simulink model "gimbal_dynamic_identification_301019"  (R2018b)
settings: Solver=FixedStepAuto  StartTime=0.0  StopTime=100  FixedStep=0.01  RelTol=1e-3
values from neighbouring files (symbols this model uses):
  DIM = data{4}    [gimbal_dynamics.m]
  DIS = data{5}    [gimbal_dynamics.m]
  I1 = data{1}    [gimbal_dynamics.m]    (also in macierze_inercji.m = sym('I1', [4 4]))
  I2 = data{2}    [gimbal_dynamics.m]    (also in macierze_inercji.m = sym('I2', [4 4]))
  I3 = data{3}    [gimbal_dynamics.m]    (also in macierze_inercji.m = sym('I3', [4 4]))
  M = [ud_ucz(3:p-1) ud_ucz(3:p-1).^2 ud_ucz(3:p-1).^3 ud_ucz(2:p-2) ud_ucz(2:p-2).^2 ud_ucz(2:p-2).^3 ud_ucz(1:p-3) ud_ucz(1:p-3).^2 ud_ucz(1:p-3).^3 yd_ucz(3:p-1) yd_ucz(3:p-1).^2 yd_ucz(3:p-1).^3 yd_ucz(2:p-2) yd_ucz(2:p-2).^2 yd_ucz(2:p-2).^3 yd_ucz(1:p-3) yd_ucz(1:p-3).^2 yd_ucz(1:p-3).^3]    [Identification_20191023.m]    (also in MI_beta.m = fillmissing(M,'spline'); gimbal_dynamics.m = data{6}; macierze_inercji.m = sym('M', [1 3]))
libraries: simulink x4, simulink_extras x3
settings Model: Creator=Paweł Tymiński  LastModifiedBy=Paweł Tymiński
settings SolverCC: ZeroCrossAlgorithm=Adaptive
settings DebuggingCC: IgnoredZcDiagnostic=none
settings SFSimCC: SimUseLocalCustomCode=off
settings RTWCC: RTWUseLocalCustomCode=off
settings CodeAppCC: StateflowObjectComments=on
settings SimscapeCC: SimscapeNormalizeSystem=off

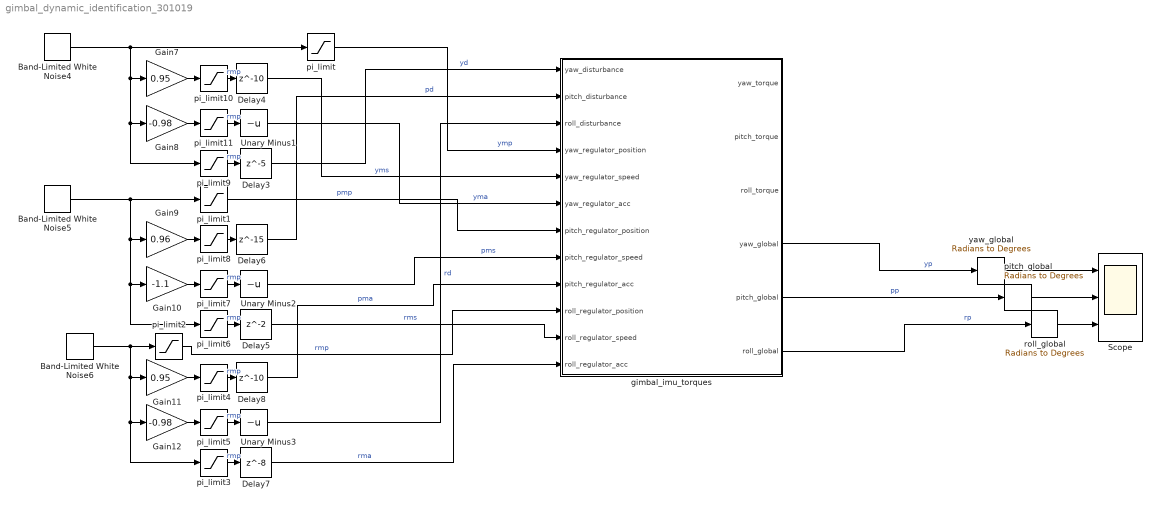
== system gimbal_dynamic_identification_301019 ==
  Band-Limited White Noise4 : simulink/Sources/Band-Limited White Noise  Cov=[0.02]  Ts=0.01  seed=[911]
  Band-Limited White Noise5 : simulink/Sources/Band-Limited White Noise  Cov=[0.015]  Ts=0.01  seed=[2137]
  Band-Limited White Noise6 : simulink/Sources/Band-Limited White Noise  Cov=[0.025]  Ts=0.01  seed=[1488]
  Delay3 : Delay  DelayLength=5  InitialCondition=0
  Delay4 : Delay  DelayLength=10  InitialCondition=0
  Delay5 : Delay  InitialCondition=0
  Delay6 : Delay  DelayLength=15  InitialCondition=0
  Delay7 : Delay  DelayLength=8  InitialCondition=0
  Delay8 : Delay  DelayLength=10  InitialCondition=0
  Gain10 : Gain  Gain=-1.1
  Gain11 : Gain  Gain=0.95
  Gain12 : Gain  Gain=-0.98
  Gain7 : Gain  Gain=0.95
  Gain8 : Gain  Gain=-0.98
  Gain9 : Gain  Gain=0.96
  Scope : Scope  NumInputPorts=3
  Unary Minus1 : UnaryMinus
  Unary Minus2 : UnaryMinus
  Unary Minus3 : UnaryMinus
  gimbal_imu_torques : Subsystem
  pi_limit{,1..11} (12 alike) : Saturate  UpperLimit=pi()  LowerLimit=-pi()
  pitch_global : simulink_extras/Transformations/Radians to Degrees
  roll_global : simulink_extras/Transformations/Radians to Degrees
  yaw_global : simulink_extras/Transformations/Radians to Degrees
  wires:
  gimbal_imu_torques/5(pitch_global) -> pitch_global/1  "pp"
  gimbal_imu_torques/4(yaw_global) -> yaw_global/1  "yp"
  gimbal_imu_torques/6(roll_global) -> roll_global/1  "rp"
  roll_global/1 -> Scope/3
  pitch_global/1 -> Scope/2
  yaw_global/1 -> Scope/1
  pi_limit/1 -> gimbal_imu_torques/4(yaw_regulator_position)  "ymp"
  Delay4/1 -> gimbal_imu_torques/5(yaw_regulator_speed)  "yms"
  pi_limit2/1 -> gimbal_imu_torques/10(roll_regulator_position)  "rmp"
  Unary Minus1/1 -> gimbal_imu_torques/6(yaw_regulator_acc)  "yma"
  Delay8/1 -> gimbal_imu_torques/9(pitch_regulator_acc)  "pma"
  pi_limit1/1 -> gimbal_imu_torques/7(pitch_regulator_position)  "pmp"
  Delay5/1 -> gimbal_imu_torques/11(roll_regulator_speed)  "rms"
  Unary Minus2/1 -> gimbal_imu_torques/8(pitch_regulator_speed)  "pms"
  Delay7/1 -> gimbal_imu_torques/12(roll_regulator_acc)  "rma"
  Band-Limited White Noise4/1 -> pi_limit9/1, Gain8/1, Gain7/1, pi_limit/1
  Band-Limited White Noise5/1 -> pi_limit6/1, Gain10/1, Gain9/1, pi_limit1/1
  Gain11/1 -> pi_limit4/1
  Gain8/1 -> pi_limit11/1
  Gain7/1 -> pi_limit10/1
  Band-Limited White Noise6/1 -> pi_limit3/1, Gain12/1, Gain11/1, pi_limit2/1
  Gain10/1 -> pi_limit7/1
  pi_limit8/1 -> Delay6/1
  Delay3/1 -> gimbal_imu_torques/1(yaw_disturbance)  "yd"
  Delay6/1 -> gimbal_imu_torques/2(pitch_disturbance)  "pd"
  Unary Minus3/1 -> gimbal_imu_torques/3(roll_disturbance)  "rd"
  pi_limit3/1 -> Delay7/1  "rmp"
  pi_limit4/1 -> Delay8/1  "rmp"
  Gain12/1 -> pi_limit5/1
  pi_limit5/1 -> Unary Minus3/1  "rmp"
  pi_limit6/1 -> Delay5/1  "rmp"
  pi_limit7/1 -> Unary Minus2/1  "rmp"
  Gain9/1 -> pi_limit8/1
  pi_limit9/1 -> Delay3/1  "rmp"
  pi_limit10/1 -> Delay4/1  "rmp"
  pi_limit11/1 -> Unary Minus1/1  "rmp"

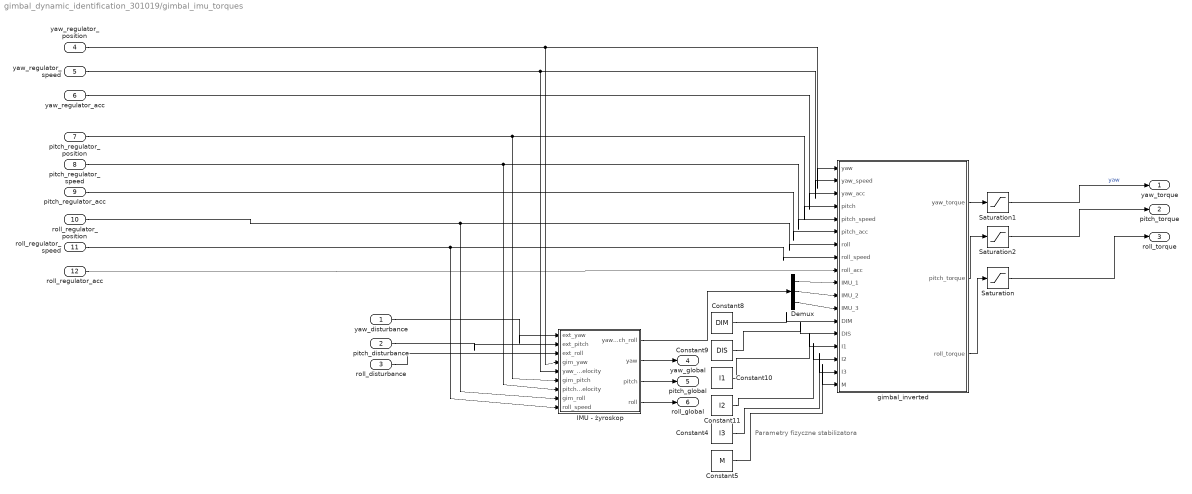
== system gimbal_dynamic_identification_301019/gimbal_imu_torques ==
  note: Parametry fizyczne stabilizatora
  yaw_disturbance : Inport
  pitch_disturbance : Inport  Port=2
  roll_disturbance : Inport  Port=3
  yaw_regulator_position : Inport  Port=4
  yaw_regulator_speed : Inport  Port=5
  yaw_regulator_acc : Inport  Port=6
  pitch_regulator_position : Inport  Port=7
  pitch_regulator_speed : Inport  Port=8
  pitch_regulator_acc : Inport  Port=9
  roll_regulator_position : Inport  Port=10
  roll_regulator_speed : Inport  Port=11
  roll_regulator_acc : Inport  Port=12
  Constant10 : Constant  Value=I1
  Constant11 : Constant  Value=I2
  Constant4 : Constant  Value=I3
  Constant5 : Constant  Value=M
  Constant8 : Constant  Value=DIM
  Constant9 : Constant  Value=DIS
  Demux : Demux  Outputs=3
  IMU - żyroskop : Subsystem
  Saturation : Saturate  UpperLimit=10  LowerLimit=-10
  Saturation1 : Saturate  UpperLimit=10  LowerLimit=-10
  Saturation2 : Saturate  UpperLimit=10  LowerLimit=-10
  gimbal_inverted : MATLAB Function  TreatAsAtomicUnit=on
  yaw_torque : Outport
  pitch_torque : Outport  Port=2
  roll_torque : Outport  Port=3
  yaw_global : Outport  Port=4
  pitch_global : Outport  Port=5
  roll_global : Outport  Port=6
  wires:
  Demux/1 -> gimbal_inverted/10(IMU_1)
  roll_regulator_position/1 -> IMU - żyroskop/8("gim_roll "), gimbal_inverted/7(roll)
  pitch_regulator_position/1 -> IMU - żyroskop/6(gim_pitch), gimbal_inverted/4(pitch)
  gimbal_inverted/2(pitch_torque) -> Saturation2/1
  yaw_regulator_speed/1 -> IMU - żyroskop/5(yaw_velocity), gimbal_inverted/2(yaw_speed)
  Demux/2 -> gimbal_inverted/11(IMU_2)
  yaw_regulator_acc/1 -> gimbal_inverted/3(yaw_acc)
  IMU - żyroskop/1(yaw_pitch_roll) -> Demux/1
  Demux/3 -> gimbal_inverted/12(IMU_3)
  roll_regulator_speed/1 -> IMU - żyroskop/9(roll_speed), gimbal_inverted/8(roll_speed)
  pitch_regulator_speed/1 -> gimbal_inverted/5(pitch_speed), IMU - żyroskop/7(pitch_velocity)
  Constant8/1 -> gimbal_inverted/13(DIM)
  Constant4/1 -> gimbal_inverted/17(I3)
  IMU - żyroskop/3(pitch) -> pitch_global/1
  gimbal_inverted/3(roll_torque) -> Saturation/1
  Constant11/1 -> gimbal_inverted/16(I2)
  Constant5/1 -> gimbal_inverted/18(M)
  gimbal_inverted/1(yaw_torque) -> Saturation1/1
  pitch_regulator_acc/1 -> gimbal_inverted/6(pitch_acc)
  Constant10/1 -> gimbal_inverted/15(I1)
  pitch_disturbance/1 -> IMU - żyroskop/2(ext_pitch)
  IMU - żyroskop/4(roll) -> roll_global/1
  IMU - żyroskop/2(yaw) -> yaw_global/1
  roll_disturbance/1 -> IMU - żyroskop/3(ext_roll)
  Constant9/1 -> gimbal_inverted/14(DIS)
  yaw_disturbance/1 -> IMU - żyroskop/1(ext_yaw)
  Saturation/1 -> roll_torque/1
  Saturation2/1 -> pitch_torque/1
  Saturation1/1 -> yaw_torque/1  "yaw"
  yaw_regulator_position/1 -> gimbal_inverted/1(yaw), IMU - żyroskop/4(gim_yaw)
  roll_regulator_acc/1 -> gimbal_inverted/9(roll_acc)

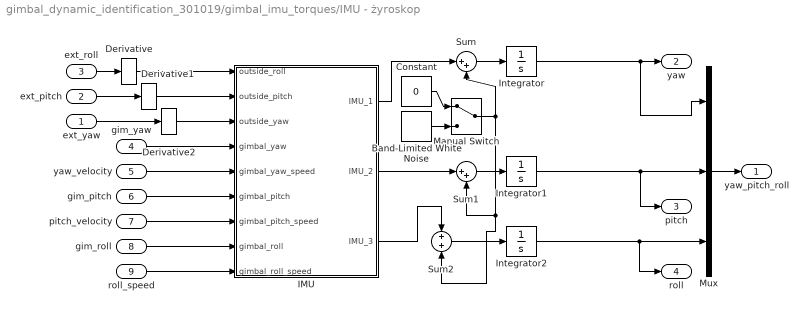
== system gimbal_dynamic_identification_301019/gimbal_imu_torques/IMU - żyroskop ==
  ext_yaw : Inport
  ext_pitch : Inport  Port=2
  ext_roll : Inport  Port=3
  gim_yaw : Inport  Port=4
  yaw_velocity : Inport  Port=5
  gim_pitch : Inport  Port=6
  pitch_velocity : Inport  Port=7
  "gim_roll " : Inport  Port=8
  roll_speed : Inport  Port=9
  Band-Limited White Noise : simulink/Sources/Band-Limited White Noise  Cov=[0.1]  Ts=0.1  seed=[23341]
  Constant : Constant  Value=0
  Derivative : Derivative
  Derivative1 : Derivative
  Derivative2 : Derivative
  IMU : MATLAB Function  TreatAsAtomicUnit=on
  Integrator : Integrator
  Integrator1 : Integrator
  Integrator2 : Integrator
  Manual Switch : ManualSwitch
  Mux : Mux  Inputs=3
  Sum : Sum  Inputs=|++
  Sum1 : Sum  Inputs=|++
  Sum2 : Sum
  yaw_pitch_roll : Outport
  yaw : Outport  Port=2
  pitch : Outport  Port=3
  roll : Outport  Port=4
  wires:
  roll_speed/1 -> IMU/9(gimbal_roll_speed)
  gim_pitch/1 -> IMU/6(gimbal_pitch)
  Mux/1 -> yaw_pitch_roll/1
  yaw_velocity/1 -> IMU/5(gimbal_yaw_speed)
  IMU/1(IMU_1) -> Sum/1
  pitch_velocity/1 -> IMU/7(gimbal_pitch_speed)
  ext_pitch/1 -> Derivative1/1
  ext_roll/1 -> Derivative/1
  ext_yaw/1 -> Derivative2/1
  "gim_roll "/1 -> IMU/8(gimbal_roll)
  gim_yaw/1 -> IMU/4(gimbal_yaw)
  IMU/3(IMU_3) -> Sum2/1
  IMU/2(IMU_2) -> Sum1/1
  Manual Switch/1 -> Sum2/2, Sum1/2, Sum/2
  Sum2/1 -> Integrator2/1
  Sum1/1 -> Integrator1/1
  Sum/1 -> Integrator/1
  Band-Limited White Noise/1 -> Manual Switch/2
  Constant/1 -> Manual Switch/1
  Derivative/1 -> IMU/1(outside_roll)
  Derivative1/1 -> IMU/2(outside_pitch)
  Derivative2/1 -> IMU/3(outside_yaw)
  Integrator/1 -> Mux/1, yaw/1
  Integrator2/1 -> roll/1, Mux/3
  Integrator1/1 -> pitch/1, Mux/2

== matlab function gimbal_dynamic_identification_301019/gimbal_imu_torques/IMU - żyroskop/IMU ==
  data: outside_roll input; IMU_1 output; outside_pitch input; outside_yaw input; gimbal_yaw input; gimbal_yaw_speed input; gimbal_pitch input; gimbal_pitch_speed input; gimbal_roll input; gimbal_roll_speed input; IMU_2 output; IMU_3 output

function [IMU_1, IMU_2, IMU_3] = IMU(outside_roll,outside_pitch,outside_yaw,gimbal_yaw ,gimbal_yaw_speed, gimbal_pitch ,gimbal_pitch_speed , gimbal_roll , gimbal_roll_speed  )
% kąty gimbala
theta_1 = gimbal_yaw ;
theta_2 = gimbal_pitch ;
theta_3 = gimbal_roll ;

J_0 =[1 0 0;
    0 cos(theta_1) -sin(theta_1);
   -sin(theta_2) cos(theta_2)*sin(theta_1) cos(theta_1)*cos(theta_2)];
Phi_0 = [outside_yaw; outside_pitch; outside_roll];

Omega_phi = J_0*Phi_0;

Omega = [gimbal_yaw_speed; gimbal_pitch_speed; gimbal_roll_speed];

J = [cos(theta_2)*cos(theta_3) sin(theta_3) 0;
    cos(theta_2)*sin(theta_3) cos(theta_3) 0;
    -sin(theta_2) 0 1];
A=J*(Omega_phi + Omega);

IMU_1 = A(1); %yaw
IMU_2 = A(2); %pitch
IMU_3 = A(3); %roll

end

== matlab function gimbal_dynamic_identification_301019/gimbal_imu_torques/gimbal_inverted ==
  data: yaw input; yaw_speed input; yaw_acc input; pitch input; pitch_speed input; pitch_acc input; roll input; yaw_torque output; roll_speed input; roll_acc input; IMU_1 input; IMU_2 input; IMU_3 input; DIM input; DIS input; I1 input; I2 input; I3 input; M input; pitch_torque output; roll_torque output
function [yaw_torque, pitch_torque, roll_torque]  = gimbal_dynamics(yaw,yaw_speed,yaw_acc,pitch,pitch_speed,pitch_acc,roll,roll_speed, roll_acc,IMU_1,IMU_2,IMU_3,DIM,DIS,I1,I2,I3,M)

%stała grawitacji
g = 9.81;


%-------------ZMIENNE--------------
% odczyty z IMU
alpha_1 = IMU_1;
alpha_2 = IMU_2;
alpha_3 = IMU_3;
IMU = [alpha_1; alpha_2; alpha_3];
%predkosci katowe osiagane przez gimbal
 om_1 = yaw_speed ;
 om_2 = pitch_speed ;
 om_3 = roll_speed ;
Omega = [om_1; om_2; om_3];
%kąty osiagane aktualnie przez gimbal
 theta_1 = yaw ;
 theta_2 = pitch ;
 theta_3 = roll ;
 THETA = [theta_1; theta_2; theta_3];
% przyśpieszenia kątowe w osiach gimbala
 ACC = [yaw_acc;pitch_acc;roll_acc];

%---------------FUNKCJE---------------------

H = calculate_H_matrix(THETA,Omega,I1,I2,I3,DIM);
D = calculate_D_matrix(THETA,I1,I2,I3,DIM);
G = calculate_G_matrix(IMU,THETA,DIM,g,M,DIS);
Q = D*ACC+H+G;
yaw_torque = Q(1);
pitch_torque = Q(2);
roll_torque = Q(3);

end
